simulink model "symodel_simple_lp"  (R2017a)
settings: Solver=FixedStepAuto  StartTime=0.0  StopTime=stoptime  FixedStep=timestep  RelTol=1e-3
undefined symbols (not defined in the file): alpha, buffer, fnoise, fseed, omega0, phi0, Plo, Prx, snoise, sseed, tau, timestep
libraries: simulink x4
settings Model: Creator=taehwan  LastModifiedBy=taehwan

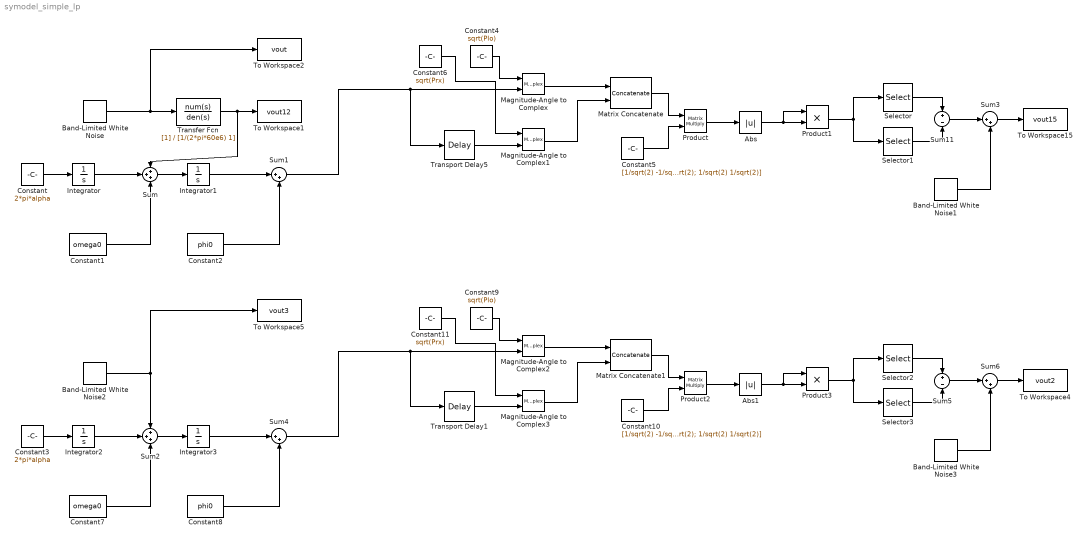
== system symodel_simple_lp ==
  Abs : Abs
  Abs1 : Abs
  Band-Limited White Noise : simulink/Sources/Band-Limited White Noise  Cov=[fnoise*2*pi]  Ts=timestep  seed=[fseed]
  Band-Limited White Noise1 : simulink/Sources/Band-Limited White Noise  Cov=[snoise]  Ts=timestep  seed=[sseed]
  Band-Limited White Noise2 : simulink/Sources/Band-Limited White Noise  Cov=[fnoise*2*pi]  Ts=timestep  seed=[fseed]
  Band-Limited White Noise3 : simulink/Sources/Band-Limited White Noise  Cov=[snoise]  Ts=timestep  seed=[sseed]
  Constant : Constant  Value=2*pi*alpha
  Constant1 : Constant  Value=omega0
  Constant10 : Constant  Value=[1/sqrt(2) -1/sqrt(2); 1/sqrt(2) 1/sqrt(2)]
  Constant11 : Constant  Value=sqrt(Prx)
  Constant2 : Constant  Value=phi0
  Constant3 : Constant  Value=2*pi*alpha
  Constant4 : Constant  Value=sqrt(Plo)
  Constant5 : Constant  Value=[1/sqrt(2) -1/sqrt(2); 1/sqrt(2) 1/sqrt(2)]
  Constant6 : Constant  Value=sqrt(Prx)
  Constant7 : Constant  Value=omega0
  Constant8 : Constant  Value=phi0
  Constant9 : Constant  Value=sqrt(Plo)
  Integrator{,1..3} (4 alike) : Integrator
  Magnitude-Angle to Complex{,1..3} (4 alike) : MagnitudeAngleToComplex
  Matrix Concatenate : Concatenate  Mode=Multidimensional array  ConcatenateDimension=2
  Matrix Concatenate1 : Concatenate  Mode=Multidimensional array  ConcatenateDimension=2
  Product : Product  Multiplication=Matrix(*)
  Product1 : Product
  Product2 : Product  Multiplication=Matrix(*)
  Product3 : Product
  Selector : Selector  InputPortWidth=2  IndexOptions=Index vector (dialog)  Indices=[1]  OutputSizes=1
  Selector1 : Selector  InputPortWidth=2  IndexOptions=Index vector (dialog)  Indices=[2]  OutputSizes=1
  Selector2 : Selector  InputPortWidth=2  IndexOptions=Index vector (dialog)  Indices=[1]  OutputSizes=1
  Selector3 : Selector  InputPortWidth=2  IndexOptions=Index vector (dialog)  Indices=[2]  OutputSizes=1
  Sum : Sum  Inputs=+++
  Sum{1,3..4,6} (4 alike) : Sum  Inputs=|++
  Sum11 : Sum  Inputs=+|-
  Sum2 : Sum  Inputs=+++
  Sum5 : Sum  Inputs=+|-
  To Workspace1 : ToWorkspace  VariableName=vout12  SaveFormat=Timeseries  SampleTime=-1
  To Workspace15 : ToWorkspace  VariableName=vout15  SaveFormat=Timeseries  SampleTime=-1
  To Workspace2 : ToWorkspace  VariableName=vout  SaveFormat=Timeseries  SampleTime=-1
  To Workspace4 : ToWorkspace  VariableName=vout2  SaveFormat=Timeseries  SampleTime=-1
  To Workspace5 : ToWorkspace  VariableName=vout3  SaveFormat=Timeseries  SampleTime=-1
  Transfer Fcn : TransferFcn  Denominator=[1/(2*pi*60e6) 1]
  Transport Delay1 : TransportDelay  DelayTime=tau  BufferSize=buffer
  Transport Delay5 : TransportDelay  DelayTime=tau  BufferSize=buffer
  wires:
  Constant/1 -> Integrator/1
  Sum/1 -> Integrator1/1
  Integrator1/1 -> Sum1/1
  Constant2/1 -> Sum1/2
  Sum1/1 -> Transport Delay5/1, Magnitude-Angle to Complex/2
  Constant1/1 -> Sum/3
  Integrator/1 -> Sum/2
  Band-Limited White Noise/1 -> To Workspace2/1, Transfer Fcn/1
  Magnitude-Angle to Complex/1 -> Matrix Concatenate/1
  Constant4/1 -> Magnitude-Angle to Complex/1
  Constant5/1 -> Product/2
  Transport Delay5/1 -> Magnitude-Angle to Complex1/2
  Matrix Concatenate/1 -> Product/1
  Product/1 -> Abs/1
  Selector/1 -> Sum11/1
  Selector1/1 -> Sum11/2
  Constant6/1 -> Magnitude-Angle to Complex1/1
  Magnitude-Angle to Complex1/1 -> Matrix Concatenate/2
  Abs/1 -> Product1/2, Product1/1
  Product1/1 -> Selector/1, Selector1/1
  Sum3/1 -> To Workspace15/1
  Sum11/1 -> Sum3/1
  Band-Limited White Noise1/1 -> Sum3/2
  Transfer Fcn/1 -> Sum/1, To Workspace1/1
  Sum2/1 -> Integrator3/1
  Constant3/1 -> Integrator2/1
  Sum4/1 -> Transport Delay1/1, Magnitude-Angle to Complex2/2
  Constant8/1 -> Sum4/2
  Integrator3/1 -> Sum4/1
  Magnitude-Angle to Complex2/1 -> Matrix Concatenate1/1
  Integrator2/1 -> Sum2/2
  Sum5/1 -> Sum6/1
  Constant10/1 -> Product2/2
  Constant9/1 -> Magnitude-Angle to Complex2/1
  Constant11/1 -> Magnitude-Angle to Complex3/1
  Constant7/1 -> Sum2/3
  Matrix Concatenate1/1 -> Product2/1
  Product2/1 -> Abs1/1
  Selector2/1 -> Sum5/1
  Transport Delay1/1 -> Magnitude-Angle to Complex3/2
  Band-Limited White Noise2/1 -> Sum2/1, To Workspace5/1
  Selector3/1 -> Sum5/2
  Abs1/1 -> Product3/2, Product3/1
  Product3/1 -> Selector2/1, Selector3/1
  Sum6/1 -> To Workspace4/1
  Magnitude-Angle to Complex3/1 -> Matrix Concatenate1/2
  Band-Limited White Noise3/1 -> Sum6/2
